simulink model "Ejercicio8_30_03_17"  (R2013a)
settings: Solver=ode23tb  StartTime=0.0  StopTime=0.5  RelTol=1e-3
libraries: powerlib x30, powerlib_meascontrol x8
settings Model: Creator=Miguel  LastModifiedBy=Miguel

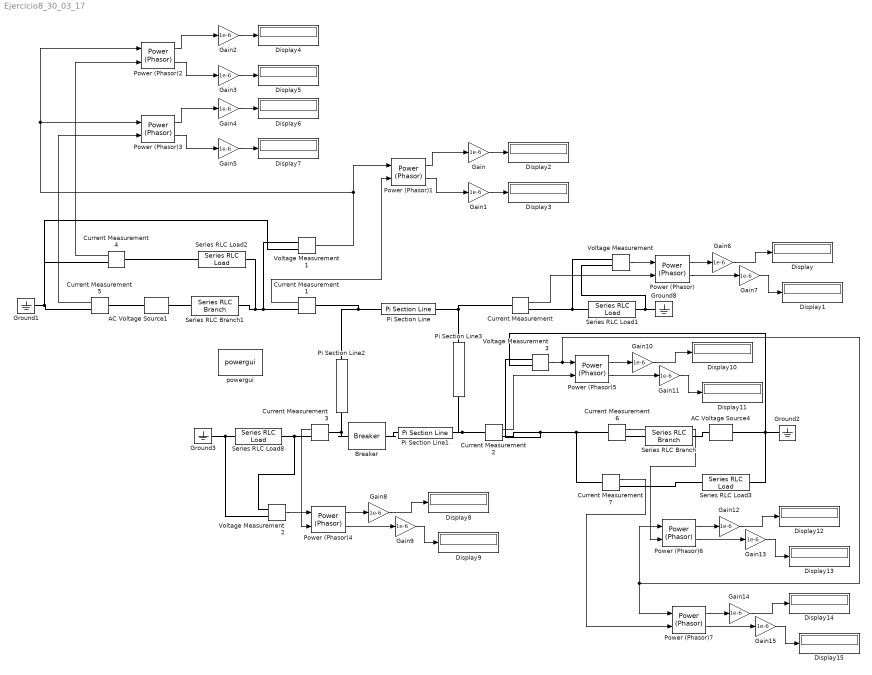
== system Ejercicio8_30_03_17 ==
  AC Voltage Source1 : powerlib/Electrical Sources/AC Voltage Source  Amplitude=150e3*sqrt(2)  Phase=0  Frequency=60  SampleTime=0  Measurements=None
  AC Voltage Source4 : powerlib/Electrical Sources/AC Voltage Source  Amplitude=1.02*sqrt(2)*150e3  Phase=1.5231  Frequency=60  SampleTime=0  Measurements=None
  Breaker : powerlib/Elements/Breaker  BreakerResistance=0.01  InitialState=0  SnubberResistance=1e6  SnubberCapacitance=inf  SwitchingTimes=[ 4/60 ]  External=off  Measurements=None  MoreParameters=off  NoBreakLoop=off
  Current Measurement{,1..7} (8 alike) : powerlib/Measurements/Current Measurement  PhasorSimulation=on  OutputType=Complex  PSBequivalent=0
  Display{,1..15} (16 alike) : Display
  Gain{,1..15} (16 alike) : Gain  Gain=1e-6
  Ground{1..3,8} (4 alike) : powerlib/Elements/Ground  LConnTagsString=a
  Pi Section Line : powerlib/Elements/Pi Section Line  LConnTagsString=__new0  RConnTagsString=__new0  Frequency=60  Resistance=0.01008*225  Inductance=0.05040/(2*pi*60)*225  Capacitance=0.05125/(pi*60*225)  Length=1  PiSections=1  Measurements=None
      settings: AttributesFormatString=\n
  Pi Section Line1 : powerlib/Elements/Pi Section Line  LConnTagsString=__new0  RConnTagsString=__new0  Frequency=60  Resistance=0.01272*225  Inductance=0.06360/(2*pi*60)*225  Capacitance=0.06375/(pi*60*225)  Length=1  PiSections=1  Measurements=None
      settings: AttributesFormatString=\n
  Pi Section Line2 : powerlib/Elements/Pi Section Line  LConnTagsString=__new0  RConnTagsString=__new0  Frequency=60  Resistance=0.00744*225  Inductance=0.03720/(2*pi*60)*225  Capacitance=0.03875/(pi*60*225)  Length=1  PiSections=1  Measurements=None
      settings: AttributesFormatString=\n
  Pi Section Line3 : powerlib/Elements/Pi Section Line  LConnTagsString=__new0  RConnTagsString=__new0  Frequency=60  Resistance=0.00744*225  Inductance=0.03720/(2*pi*60)*225  Capacitance=0.03875/(pi*60*225)  Length=1  PiSections=1  Measurements=None
      settings: AttributesFormatString=\n
  Power (Phasor){,1..7} (8 alike) : powerlib_meascontrol/Measurements/Power (Phasor)
  Series RLC Branch : powerlib/Elements/Series RLC Branch  LConnTagsString=__new0  RConnTagsString=__new0  BranchType=R  Resistance=1e-9  Inductance=1e-3  SetiL0=off  InitialCurrent=0  Capacitance=1e-6  Setx0=off  InitialVoltage=0  Measurements=None
  Series RLC Branch1 : powerlib/Elements/Series RLC Branch  LConnTagsString=__new0  RConnTagsString=__new0  BranchType=R  Resistance=1e-9  Inductance=1e-3  SetiL0=off  InitialCurrent=0  Capacitance=1e-6  Setx0=off  InitialVoltage=0  Measurements=None
  Series RLC Load1 : powerlib/Elements/Series RLC Load  LConnTagsString=a  RConnTagsString=__new0  NominalVoltage=0.9824*150e3  NominalFrequency=60  ActivePower=170e6  InductivePower=105.35e6  CapacitivePower=0  Setx0=off  InitialVoltage=0  SetiL0=off  InitialCurrent=0  Measurements=None
  Series RLC Load2 : powerlib/Elements/Series RLC Load  LConnTagsString=a  RConnTagsString=__new0  NominalVoltage=150e3  NominalFrequency=60  ActivePower=50e6  InductivePower=30.99e6  CapacitivePower=0  Setx0=off  InitialVoltage=0  SetiL0=off  InitialCurrent=0  Measurements=None
  Series RLC Load3 : powerlib/Elements/Series RLC Load  LConnTagsString=a  RConnTagsString=__new0  NominalVoltage=1.02*150e3  NominalFrequency=60  ActivePower=80e6  InductivePower=49.59e6  CapacitivePower=0  Setx0=off  InitialVoltage=0  SetiL0=off  InitialCurrent=0  Measurements=None
  Series RLC Load8 : powerlib/Elements/Series RLC Load  LConnTagsString=a  RConnTagsString=__new0  NominalVoltage=0.9690*150e3  NominalFrequency=60  ActivePower=200e6  InductivePower=123.94e6  CapacitivePower=0  Setx0=off  InitialVoltage=0  SetiL0=off  InitialCurrent=0  Measurements=Branch current
  Voltage Measurement{,1..3} (4 alike) : powerlib/Measurements/Voltage Measurement  PhasorSimulation=on  OutputType=Complex  PSBequivalent=0
  powergui : powerlib/powergui  Priority=1  SimulationMode=Phasor  SolverType=Tustin  SampleTime=50e-6  frequency=60  SPID=off  DisableSnubberDevices=off  DisableRonSwitches=off  DisableVfSwitches=off  SwTol=0  Interpol=off  DisplayEquations=off  frequencyindice=60  Pbase=100e6  ErrMax=1e-4  Iterations=50  UnitsV=kV  UnitsW=MW  FunctionMessages=off  echomessages=off  HookPort=off  EnableUseOfTLC=off  x0status=blocks  RestoreLinks=warning  ResistiveCurrentMeasurement=off  Frange=[0:2:500]  Ylog=off  Xlog=on  ShowGrid=off  save=off  variable=ZData  ZoomFFT=off  StartTime=0.0  cycles=1  DisplayStyle=1  fundamental=60  FreqAxis=off  MaxFrequency=1000  frequencyindicesteady=1  RmsSteady=2  display=off  Ts=0  methode=off
  wires:
  Power (Phasor)/1 -> Gain6/1
  Power (Phasor)/2 -> Gain7/1
  Voltage Measurement/1 -> Power (Phasor)/1
  Current Measurement/1 -> Power (Phasor)/2
  Power (Phasor)1/1 -> Gain/1
  Power (Phasor)1/2 -> Gain1/1
  Current Measurement1/1 -> Power (Phasor)1/2
  Gain1/1 -> Display3/1
  Gain/1 -> Display2/1
  Power (Phasor)2/1 -> Gain2/1
  Power (Phasor)2/2 -> Gain3/1
  Gain3/1 -> Display5/1
  Gain2/1 -> Display4/1
  Power (Phasor)3/1 -> Gain4/1
  Power (Phasor)3/2 -> Gain5/1
  Gain5/1 -> Display7/1
  Gain4/1 -> Display6/1
  Voltage Measurement1/1 -> Power (Phasor)1/1, Power (Phasor)2/1, Power (Phasor)3/1
  Current Measurement4/1 -> Power (Phasor)2/2
  Current Measurement5/1 -> Power (Phasor)3/2
  Gain6/1 -> Display/1
  Gain7/1 -> Display1/1
  Power (Phasor)4/1 -> Gain8/1
  Power (Phasor)4/2 -> Gain9/1
  Voltage Measurement2/1 -> Power (Phasor)4/1
  Current Measurement3/1 -> Power (Phasor)4/2
  Gain8/1 -> Display8/1
  Gain9/1 -> Display9/1
  Power (Phasor)5/1 -> Gain10/1
  Power (Phasor)5/2 -> Gain11/1
  Gain10/1 -> Display10/1
  Gain11/1 -> Display11/1
  Power (Phasor)6/1 -> Gain12/1
  Power (Phasor)6/2 -> Gain13/1
  Gain12/1 -> Display12/1
  Gain13/1 -> Display13/1
  Power (Phasor)7/1 -> Gain14/1
  Power (Phasor)7/2 -> Gain15/1
  Voltage Measurement3/1 -> Power (Phasor)7/1, Power (Phasor)6/1, Power (Phasor)5/1
  Gain14/1 -> Display14/1
  Gain15/1 -> Display15/1
  Current Measurement2/1 -> Power (Phasor)5/2
  Current Measurement6/1 -> Power (Phasor)6/2
  Current Measurement7/1 -> Power (Phasor)7/2
  connections:
  Current Measurement5/RConn1 -- Current Measurement4/RConn1 -- Voltage Measurement1/LConn2 -- Ground1/LConn1
  Current Measurement3/LConn1 -- Breaker/LConn1 -- Pi Section Line2/RConn1
  Series RLC Load1/LConn1 -- Current Measurement/RConn1 -- Voltage Measurement/LConn1
  Pi Section Line3/RConn1 -- Current Measurement2/LConn1 -- Pi Section Line1/RConn1
  Ground2/LConn1 -- Voltage Measurement3/LConn2 -- Series RLC Load3/RConn1 -- AC Voltage Source4/LConn1
  Series RLC Load8/RConn1 -- Voltage Measurement2/LConn2 -- Ground3/LConn1
  Ground8/LConn1 -- Voltage Measurement/LConn2 -- Series RLC Load1/RConn1
  Voltage Measurement1/LConn1 -- Series RLC Load2/LConn1 -- Series RLC Branch1/RConn1 -- Current Measurement1/RConn1
  Series RLC Branch1/LConn1 -- AC Voltage Source1/RConn1
  Pi Section Line3/LConn1 -- Current Measurement/LConn1 -- Pi Section Line/RConn1
  Current Measurement1/LConn1 -- Pi Section Line2/LConn1 -- Pi Section Line/LConn1
  Current Measurement3/RConn1 -- Voltage Measurement2/LConn1 -- Series RLC Load8/LConn1
  Current Measurement7/LConn1 -- Current Measurement6/LConn1 -- Voltage Measurement3/LConn1 -- Current Measurement2/RConn1
  Current Measurement5/LConn1 -- AC Voltage Source1/LConn1
  Current Measurement4/LConn1 -- Series RLC Load2/RConn1
  Series RLC Load3/LConn1 -- Current Measurement7/RConn1
  Series RLC Branch/LConn1 -- Current Measurement6/RConn1
  Series RLC Branch/RConn1 -- AC Voltage Source4/RConn1
  Breaker/RConn1 -- Pi Section Line1/LConn1
